simulink model "ChkPwrMding"  (Simulink 7.8)
settings: Solver=ode45  StartTime=0.0  StopTime=10.0  RelTol=1e-3
undefined symbols (not defined in the file): CeSTMR_e_LVR_N, CeSTMR_e_LVR_P, KeASMR_b_CheckParkAndNeutral, KeASMR_b_StrtCntrlOffChkEnbl
libraries: ChryslerLib x2
settings Model: Creator=T6684MB  LastModifiedBy=T6684MB

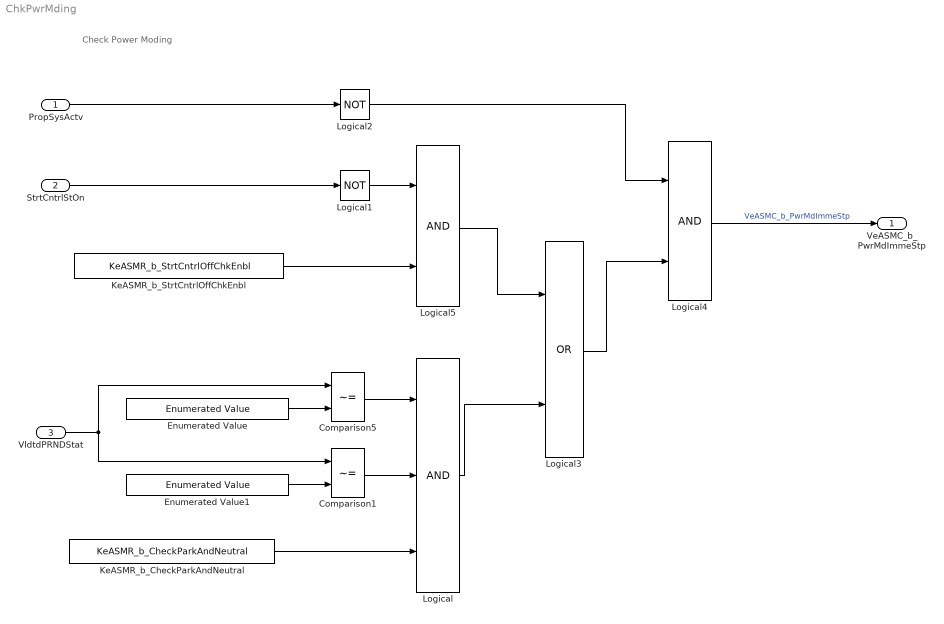
== system ChkPwrMding ==
  note: Check Power Moding
  PropSysActv : Inport
  StrtCntrlStOn : Inport  Port=2
  VldtdPRNDStat : Inport  Port=3
  Comparison1 : RelationalOperator  Operator=~=  OutDataTypeStr=boolean
  Comparison5 : RelationalOperator  Operator=~=  OutDataTypeStr=boolean
  Enumerated Value : ChryslerLib/Parameters & Constants/Enumerated Value  Value=CeSTMR_e_LVR_P  OutMin=[]  OutMax=[]  OutDataTypeStr=TeSTMR_e_Lv2PRND_Stat
  Enumerated Value1 : ChryslerLib/Parameters & Constants/Enumerated Value  Value=CeSTMR_e_LVR_N  OutMin=[]  OutMax=[]  OutDataTypeStr=TeSTMR_e_Lv2PRND_Stat
  KeASMR_b_CheckParkAndNeutral : Constant  Value=KeASMR_b_CheckParkAndNeutral
      settings: CopyFcn=try,set_param(gcb,'Value',get_param(gcb,'Name'));catch,err=lasterror;if (isempty(strfind(err.message,'Attempting to override parameters')) || isempty(strfind(err.message,'which is inside a library link'))) rethrow(err);end;end  NameChangeFcn=try,set_param(gcb,'Value',get_param(gcb,'Name'));catch,[msgstr msgid]=lasterr;errordlg(['error ',num2str(msgid),' - ',msgstr],'Error','modal');end  OpenFcn=global edelemcal; edelemcal.cb = gcb; edfigelemcal('fig');
  KeASMR_b_StrtCntrlOffChkEnbl : Constant  Value=KeASMR_b_StrtCntrlOffChkEnbl
      settings: CopyFcn=try,set_param(gcb,'Value',get_param(gcb,'Name'));catch,err=lasterror;if (isempty(strfind(err.message,'Attempting to override parameters')) || isempty(strfind(err.message,'which is inside a library link'))) rethrow(err);end;end  NameChangeFcn=try,set_param(gcb,'Value',get_param(gcb,'Name'));catch,[msgstr msgid]=lasterr;errordlg(['error ',num2str(msgid),' - ',msgstr],'Error','modal');end  OpenFcn=global edelemcal; edelemcal.cb = gcb; edfigelemcal('fig');
  Logical : Logic  Inputs=3  OutDataTypeStr=boolean
  Logical1 : Logic  Operator=NOT  OutDataTypeStr=boolean
  Logical2 : Logic  Operator=NOT  OutDataTypeStr=boolean
  Logical3 : Logic  Operator=OR  OutDataTypeStr=boolean
  Logical4 : Logic  OutDataTypeStr=boolean
  Logical5 : Logic  OutDataTypeStr=boolean
  VeASMC_b_PwrMdImmeStp : Outport
  wires:
  KeASMR_b_StrtCntrlOffChkEnbl/1 -> Logical5/2
  Logical1/1 -> Logical5/1
  Logical/1 -> Logical3/2
  Logical5/1 -> Logical3/1
  Logical3/1 -> Logical4/2
  Logical4/1 -> VeASMC_b_PwrMdImmeStp/1  "VeASMC_b_PwrMdImmeStp"
  KeASMR_b_CheckParkAndNeutral/1 -> Logical/3
  StrtCntrlStOn/1 -> Logical1/1
  Comparison1/1 -> Logical/2
  Comparison5/1 -> Logical/1
  Logical2/1 -> Logical4/1
  PropSysActv/1 -> Logical2/1
  Enumerated Value1/1 -> Comparison1/2
  VldtdPRNDStat/1 -> Comparison5/1, Comparison1/1
  Enumerated Value/1 -> Comparison5/2
